simulink library "engine_T2_lib"  (Simulink 6.6)
undefined symbols (not defined in the file): engl_ang, engr_ang
libraries: aeroutilslib x3, simulink x3, engine_JetCatP70_lib x2
settings Model: Creator=amurch  LastModifiedBy=amurch

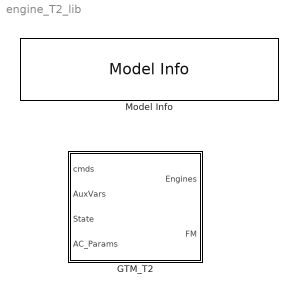
== system engine_T2_lib ==
  GTM_T2 : Subsystem
  Model Info : simulink/Model-Wide Utilities/Model Info  SystemSampleTime=-1  InitialBlockCM=None  BlockCM=None  Frame=on  DisplayStringWithTags=|  HorizontalTextAlignment=Center  LeftAlignmentValue=0.5  SourceBlockDiagram=engine_T2_lib  TagMaxNumber=20
      | GTM T2 Engine Library
      | 
      | Model Version: %<ModelVersion>
      | Last modifed by %<LastModifiedBy> on %<LastModificationDate>

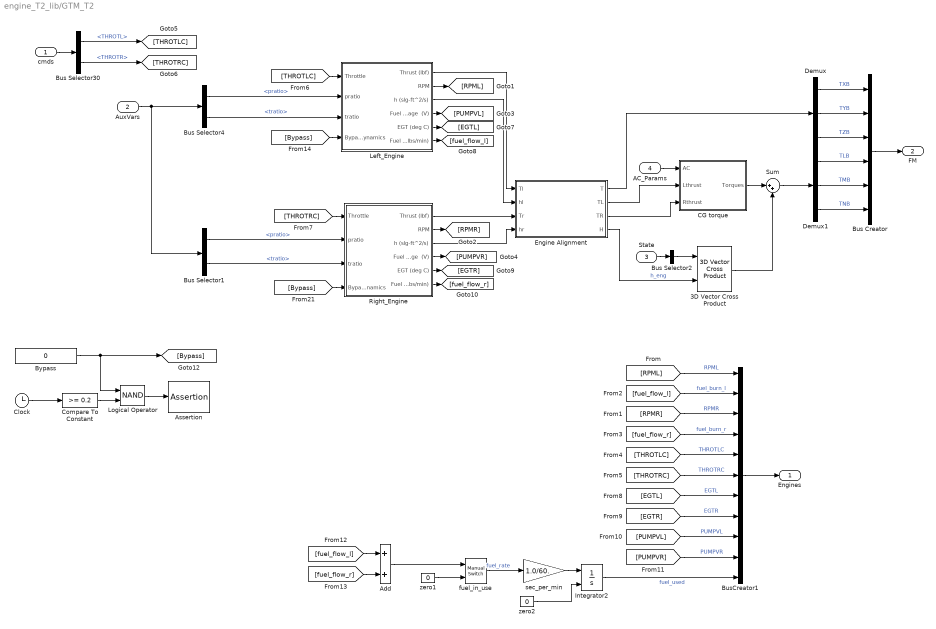
== system engine_T2_lib/GTM_T2 ==
  cmds : Inport
  AuxVars : Inport  Port=2
  State : Inport  Port=3
  AC_Params : Inport  Port=4
  3D Vector Cross Product : aeroutilslib/3D Vector Cross Product  SystemSampleTime=-1
  Add : Sum  OutScaling=2^-10
  Assertion : Assertion  Enabled=on  AssertionFailFcn=warndlg('Engine dynamics in bypass mode. Run setup.m to reset.','Warning!')
  Bus Creator : BusCreator  Inputs=6
  Bus Selector1 : BusSelector  OutputSignals=pratio,tratio
  Bus Selector2 : BusSelector  OutputSignals=pb,qb,rb  OutputAsBus=on
  Bus Selector30 : BusSelector  OutputSignals=THROTL,THROTR
  Bus Selector4 : BusSelector  OutputSignals=pratio,tratio
  BusCreator1 : BusCreator  Inputs=11
  Bypass : Constant  Value=0
  CG torque : Subsystem
  Clock : Clock
      settings: Decimation=10
  Compare To Constant : simulink/Logic and Bit Operations/Compare To Constant  SystemSampleTime=-1  relop=>=  const=0.2  LogicOutDataTypeMode=boolean  ZeroCross=off
  Demux : Demux  Outputs=3
  Demux1 : Demux  Outputs=3
  Engine Alignment : Stateflow chart
  Integrator2 : Integrator  InitialConditionSource=external
  Left_Engine : Subsystem  BlockChoice=Jetcat P70
      settings: AttributesFormatString=%<BlockChoice>  TemplateBlock=enginelib/Engine Model  MemberBlocks=AMT-180,AMT-280,Blank,Jetcat P120SE,Jetcat P70
  Logical Operator : Logic  Operator=NAND  AllPortsSameDT=off  OutDataTypeMode=Boolean
  Right_Engine : Subsystem  BlockChoice=Jetcat P70
      settings: AttributesFormatString=%<BlockChoice>  TemplateBlock=enginelib/Engine Model  MemberBlocks=AMT-180,AMT-280,Blank,Jetcat P120SE,Jetcat P70
  Sum : Sum  Inputs=|++
  fuel_in_use : simulink/Signal Routing/Manual Switch  SystemSampleTime=-1  sw=0  action=0  varsize=off
  sec_per_min : Gain  Gain=1.0/60.  SaturateOnIntegerOverflow=on
  zero1 : Constant  Value=0
  zero2 : Constant  Value=0
  Engines : Outport
  FM : Outport  Port=2  PortDimensions=6
  wires:
  Right_Engine/6(Fuel Flow (lbs/min)) -> [fuel_flow_r]
  Right_Engine/5(EGT (deg C)) -> [EGTR]
  Left_Engine/6(Fuel Flow (lbs/min)) -> [fuel_flow_l]
  Left_Engine/5(EGT (deg C)) -> [EGTL]
  cmds/1 -> Bus Selector30/1
  Demux/2 -> Bus Creator/2  "TYB"
  State/1 -> Bus Selector2/1
  Bus Selector2/1 -> 3D Vector Cross Product/1
  Demux/3 -> Bus Creator/3  "TZB"
  Left_Engine/2(RPM) -> [RPML]
  Left_Engine/4(Fuel Pump Voltage  (V)) -> [PUMPVL]
  Right_Engine/4(Fuel Pump Voltage  (V)) -> [PUMPVR]
  Right_Engine/2(RPM) -> [RPMR]
  Bus Selector1/1 -> Right_Engine/2(pratio)  "<pratio>"
  Bus Selector1/2 -> Right_Engine/3(tratio)  "<tratio>"
  AuxVars/1 -> Bus Selector1/1, Bus Selector4/1
  AC_Params/1 -> CG torque/1(AC)
  Bus Creator/1 -> FM/1
  Bus Selector30/1 -> [THROTLC]  "<THROTL>"
  Bus Selector30/2 -> [THROTRC]  "<THROTR>"
  [THROTLC] -> Left_Engine/1(Throttle)
  [THROTRC] -> Right_Engine/1(Throttle)
  [THROTRC] -> BusCreator1/6  "THROTRC"
  [THROTLC] -> BusCreator1/5  "THROTLC"
  [fuel_flow_r] -> BusCreator1/4  "fuel_burn_r"
  [fuel_flow_l] -> BusCreator1/2  "fuel_burn_l"
  [RPMR] -> BusCreator1/3  "RPMR"
  [RPML] -> BusCreator1/1  "RPML"
  BusCreator1/1 -> Engines/1
  [EGTL] -> BusCreator1/7  "EGTL"
  [EGTR] -> BusCreator1/8  "EGTR"
  [PUMPVL] -> BusCreator1/9  "PUMPVL"
  [PUMPVR] -> BusCreator1/10  "PUMPVR"
  sec_per_min/1 -> Integrator2/1
  fuel_in_use/1 -> sec_per_min/1  "fuel_rate"
  Integrator2/1 -> BusCreator1/11  "fuel_used"
  zero2/1 -> Integrator2/2
  [fuel_flow_l] -> Add/1
  [fuel_flow_r] -> Add/2
  zero1/1 -> fuel_in_use/2
  Add/1 -> fuel_in_use/1
  Bus Selector4/1 -> Left_Engine/2(pratio)  "<pratio>"
  Bus Selector4/2 -> Left_Engine/3(tratio)  "<tratio>"
  [Bypass] -> Left_Engine/4(BypassDynamics)
  [Bypass] -> Right_Engine/4(BypassDynamics)
  Bypass/1 -> Logical Operator/1, [Bypass]
  Clock/1 -> Compare To Constant/1
  Left_Engine/1(Thrust (lbf)) -> Engine Alignment/1(Tl)
  Right_Engine/1(Thrust (lbf)) -> Engine Alignment/3(Tr)
  Demux/1 -> Bus Creator/1  "TXB"
  Left_Engine/3(h (slg-ft^2/s)) -> Engine Alignment/2(hl)
  Right_Engine/3(h (slg-ft^2/s)) -> Engine Alignment/4(hr)
  Engine Alignment/4(H) -> 3D Vector Cross Product/2  "h_eng"
  Engine Alignment/1(T) -> Demux/1
  Engine Alignment/2(TL) -> CG torque/2(Lthrust)
  Engine Alignment/3(TR) -> CG torque/3(Rthrust)
  CG torque/1(Torques) -> Sum/1
  3D Vector Cross Product/1 -> Sum/2
  Sum/1 -> Demux1/1
  Demux1/1 -> Bus Creator/4  "TLB"
  Demux1/2 -> Bus Creator/5  "TMB"
  Demux1/3 -> Bus Creator/6  "TNB"
  Compare To Constant/1 -> Logical Operator/2
  Logical Operator/1 -> Assertion/1

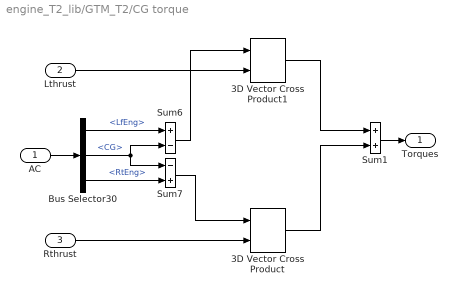
== system engine_T2_lib/GTM_T2/CG torque ==
  AC : Inport
  Lthrust : Inport  Port=2
  Rthrust : Inport  Port=3
  3D Vector Cross Product : aeroutilslib/3D Vector Cross Product  SystemSampleTime=-1
  3D Vector Cross Product1 : aeroutilslib/3D Vector Cross Product  SystemSampleTime=-1
  Bus Selector30 : BusSelector  OutputSignals=LfEng,CG,RtEng
  Sum1 : Sum  SaturateOnIntegerOverflow=on  InputSameDT=on
  Sum6 : Sum  Inputs=+-  SaturateOnIntegerOverflow=on  InputSameDT=on
  Sum7 : Sum  Inputs=-+  SaturateOnIntegerOverflow=on  InputSameDT=on
  Torques : Outport
  wires:
  AC/1 -> Bus Selector30/1
  Bus Selector30/2 -> Sum7/1, Sum6/2  "<CG>"
  Lthrust/1 -> 3D Vector Cross Product1/2
  Rthrust/1 -> 3D Vector Cross Product/2
  Sum7/1 -> 3D Vector Cross Product/1
  Sum6/1 -> 3D Vector Cross Product1/1
  3D Vector Cross Product1/1 -> Sum1/1
  3D Vector Cross Product/1 -> Sum1/2
  Sum1/1 -> Torques/1
  Bus Selector30/3 -> Sum7/2  "<RtEng>"
  Bus Selector30/1 -> Sum6/1  "<LfEng>"

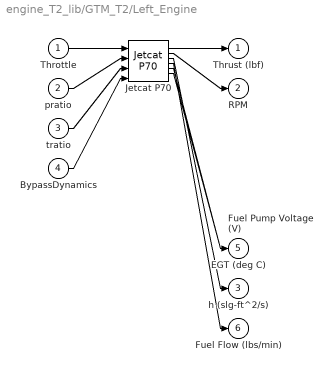
== system engine_T2_lib/GTM_T2/Left_Engine ==
  Throttle : Inport
  pratio : Inport  Port=2
  tratio : Inport  Port=3
  BypassDynamics : Inport  Port=4
  Jetcat P70 : engine_JetCatP70_lib/Jetcat P70  SystemSampleTime=-1
  Thrust (lbf) : Outport
  RPM : Outport  Port=2
  h (slg-ft^2/s) : Outport  Port=3
  Fuel Pump Voltage  (V) : Outport  Port=4
  EGT (deg C) : Outport  Port=5
  Fuel Flow (lbs/min) : Outport  Port=6
  wires:
  Throttle/1 -> Jetcat P70/1
  pratio/1 -> Jetcat P70/2
  tratio/1 -> Jetcat P70/3
  BypassDynamics/1 -> Jetcat P70/4
  Jetcat P70/1 -> Thrust (lbf)/1
  Jetcat P70/2 -> RPM/1
  Jetcat P70/3 -> h (slg-ft^2/s)/1
  Jetcat P70/4 -> Fuel Flow (lbs/min)/1
  Jetcat P70/5 -> Fuel Pump Voltage  (V)/1
  Jetcat P70/6 -> EGT (deg C)/1

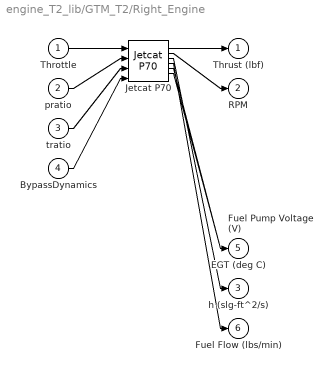
== system engine_T2_lib/GTM_T2/Right_Engine ==
  Throttle : Inport
  pratio : Inport  Port=2
  tratio : Inport  Port=3
  BypassDynamics : Inport  Port=4
  Jetcat P70 : engine_JetCatP70_lib/Jetcat P70  SystemSampleTime=-1
  Thrust (lbf) : Outport
  RPM : Outport  Port=2
  h (slg-ft^2/s) : Outport  Port=3
  Fuel Pump Voltage  (V) : Outport  Port=4
  EGT (deg C) : Outport  Port=5
  Fuel Flow (lbs/min) : Outport  Port=6
  wires:
  Throttle/1 -> Jetcat P70/1
  pratio/1 -> Jetcat P70/2
  tratio/1 -> Jetcat P70/3
  BypassDynamics/1 -> Jetcat P70/4
  Jetcat P70/1 -> Thrust (lbf)/1
  Jetcat P70/2 -> RPM/1
  Jetcat P70/3 -> h (slg-ft^2/s)/1
  Jetcat P70/4 -> Fuel Flow (lbs/min)/1
  Jetcat P70/5 -> Fuel Pump Voltage  (V)/1
  Jetcat P70/6 -> EGT (deg C)/1

== matlab function GTM_T2/Engine Alignment ==
  data: T output inherited; Tl input inherited; hl input inherited; Tr input inherited; hr input inherited; TL output inherited; engl_ang parameter inherited; engr_ang parameter inherited; TR output inherited; H output inherited
function [T,TL,TR,H] = eng_angles(Tl,hl,Tr,hr,engl_ang,engr_ang)
% This block supports an embeddable subset of the MATLAB language.
% See the help menu for details. 

% Using the engine alignment angles (set in AC_params_T2.m), compute the 
% off-axis thrust and angular momentum terms.

TL = Tl*[cosd(engl_ang(2))*cosd(engl_ang(3));...
         -sind(engl_ang(3));...
         sind(engl_ang(2))*cosd(engl_ang(3))];
TR = Tr*[cosd(engr_ang(2))*cosd(engr_ang(3));...
         -sind(engr_ang(3));...
         sind(engr_ang(2))*cosd(engr_ang(3))];  
T = TL+TR;

H = hl*[cosd(engl_ang(2))*cosd(engl_ang(3));...
         -sind(engl_ang(3));...
         sind(engl_ang(2))*cosd(engl_ang(3))] + ...
         hr*[cosd(engr_ang(2))*cosd(engr_ang(3));...
         -sind(engr_ang(3));...
         sind(engr_ang(2))*cosd(engr_ang(3))];
